simulink model "encoder_quantizer"  (R2015a)
settings: Solver=ode45  StartTime=0.0  StopTime=10.0  RelTol=1e-3
libraries: dspquant2 x1
settings Model: Creator=preston  LastModifiedBy=Nathan

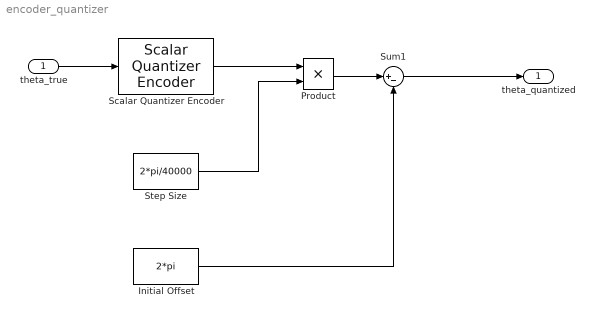
== system encoder_quantizer ==
  theta_true : Inport
  Initial Offset : Constant  Value=2*pi
  Product : Product
  Scalar Quantizer Encoder : dspquant2/Scalar Quantizer Encoder  paramSrc=Specify via dialog  partType=Bounded  BBoundary=[-2*pi:2*pi/40000:2*pi]  UBoundary=[2:9]  SearchMethod=Binary  tieBreakRule=Choose the lower index  outQU=off  outQError=off  codebook=[-2*pi+pi/10000:2*pi/10000:2*pi]  outStatus=off  invalidin=Clip and warn  idtype=int32  roundingMode=Floor  overflowMode=off
  Step Size : Constant  Value=2*pi/40000
  Sum1 : Sum  Inputs=|+-
  theta_quantized : Outport
  wires:
  theta_true/1 -> Scalar Quantizer Encoder/1
  Scalar Quantizer Encoder/1 -> Product/1
  Step Size/1 -> Product/2
  Product/1 -> Sum1/1
  Initial Offset/1 -> Sum1/2
  Sum1/1 -> theta_quantized/1
